simulink model "HF_simulink"  (R2017a)
settings: Solver=VariableStepAuto  StartTime=0.0  StopTime=60  RelTol=1e-3
values from neighbouring files (symbols this model uses):
  g = 9.8    [Coeficientes.mat]
  Iyy = 0.0191    [Coeficientes.mat]
  l1 = 0.25    [Coeficientes.mat]
  m = 0.8    [Coeficientes.mat]
settings Model: Creator=ferra  LastModifiedBy=ferra

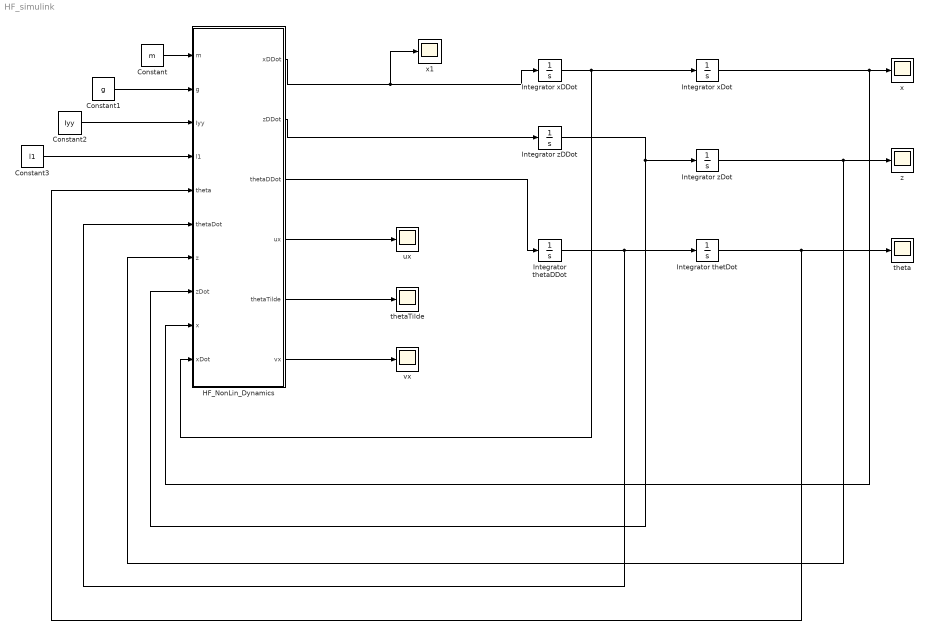
== system HF_simulink ==
  Constant : Constant  Value=m
  Constant1 : Constant  Value=g
  Constant2 : Constant  Value=Iyy
  Constant3 : Constant  Value=l1
  "HF_NonLin_Dynamics " : MATLAB Function  TreatAsAtomicUnit=on
  Integrator thetDot : Integrator  InitialCondition=pi/8
  Integrator thetaDDot : Integrator
  Integrator xDDot : Integrator
  "Integrator xDot " : Integrator  InitialCondition=2
  Integrator zDDot : Integrator
  Integrator zDot : Integrator
  theta : Scope
  thetaTilde : Scope
  ux : Scope
  vx : Scope
  x : Scope
  x1 : Scope
  z : Scope
  wires:
  "HF_NonLin_Dynamics "/1(xDDot) -> x1/1, Integrator xDDot/1
  Integrator xDDot/1 -> "HF_NonLin_Dynamics "/10(xDot), "Integrator xDot "/1
  "Integrator xDot "/1 -> "HF_NonLin_Dynamics "/9(x), x/1
  "HF_NonLin_Dynamics "/2(zDDot) -> Integrator zDDot/1
  Integrator zDot/1 -> "HF_NonLin_Dynamics "/7(z), z/1
  Integrator zDDot/1 -> "HF_NonLin_Dynamics "/8(zDot), Integrator zDot/1
  Integrator thetaDDot/1 -> "HF_NonLin_Dynamics "/6(thetaDot), Integrator thetDot/1
  Integrator thetDot/1 -> "HF_NonLin_Dynamics "/5(theta), theta/1
  Constant/1 -> "HF_NonLin_Dynamics "/1(m)
  Constant1/1 -> "HF_NonLin_Dynamics "/2(g)
  Constant2/1 -> "HF_NonLin_Dynamics "/3(Iyy)
  Constant3/1 -> "HF_NonLin_Dynamics "/4(l1)
  "HF_NonLin_Dynamics "/3(thetaDDot) -> Integrator thetaDDot/1
  "HF_NonLin_Dynamics "/5(thetaTilde) -> thetaTilde/1
  "HF_NonLin_Dynamics "/4(ux) -> ux/1
  "HF_NonLin_Dynamics "/6(vx) -> vx/1

== matlab function HF_simulink/HF_NonLin_Dynamics  ==
  data: m input; g input; Iyy input; l1 input; theta input; thetaDot input; xDDot output; zDDot output; thetaDDot output; z input; zDot input; x input; xDot input; ux output; thetaTilde output; vx output
function [xDDot,zDDot,thetaDDot,ux,thetaTilde,vx] = HF_NonLin_Dynamics(m,g,Iyy,l1,theta,thetaDot,z,zDot,x,xDot)

Kpz = 3;
Kdz = 3;

Kpx = 2;
Kdx = 1.2;

zDes = -8;
xDes = 4;
uz = -Kpz * (z - zDes) - Kdz * zDot;

vx =  -Kpx * (x-xDes) -Kdx * xDot;

ux = atan(-vx/g);

thetaTilde = theta - ux ;

Tt = -(m*uz - m*g)/(cos(theta));
Td = (tanh(thetaTilde) + tanh(thetaDot))/l1;


% xDDot = -(Tt * sin(ux))/m ;
xDDot = -g * tan(ux);
zDDot = -(Tt*cos(theta))/m + g;
thetaDDot = -(l1 * Td)/Iyy;
end
